simulink model "manning_weir_nonlinear"  (R2022b)
settings: Solver=VariableStepAuto  StartTime=0.0  StopTime=5*N  RelTol=1e-3
libraries: cstblocks x3
settings Model: Creator=chuan  LastModifiedBy=chuan

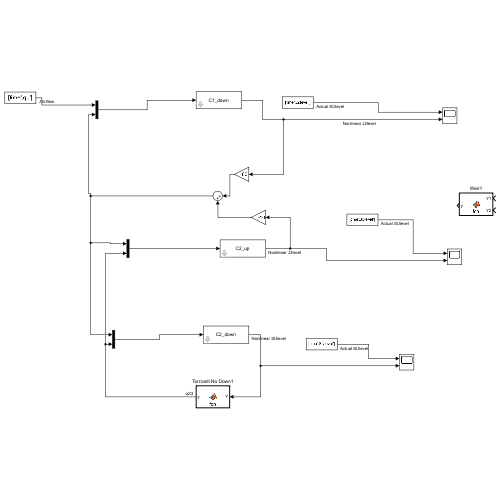
[thumbnail: Simulink's stored preview of the top-level diagram]
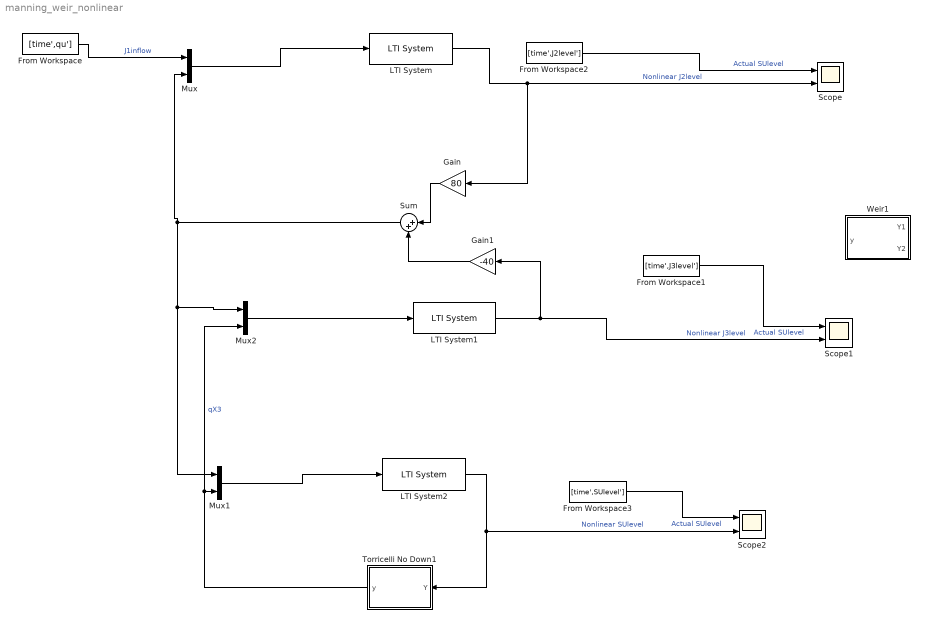
== system manning_weir_nonlinear ==
  From Workspace : FromWorkspace  VariableName=[time',qu']
  From Workspace1 : FromWorkspace  VariableName=[time',J3level']
  From Workspace2 : FromWorkspace  VariableName=[time',J2level']
  From Workspace3 : FromWorkspace  VariableName=[time',SUlevel']
  Gain : Gain  Gain=80
  Gain1 : Gain  Gain=-40
  LTI System : cstblocks/LTI System  sys=C1_down  IC=[]
  LTI System1 : cstblocks/LTI System  sys=C2_up  IC=[]
  LTI System2 : cstblocks/LTI System  sys=C2_down  IC=[]
  Mux : Mux  Inputs=2
  Mux1 : Mux  Inputs=2
  Mux2 : Mux  Inputs=2
  Scope : Scope  NumInputPorts=2
  Scope1 : Scope  NumInputPorts=2
  Scope2 : Scope  NumInputPorts=2
  Sum : Sum  Inputs=|++
  Torricelli No Down1 : MATLAB Function  TreatAsAtomicUnit=on
  Weir1 : MATLAB Function  TreatAsAtomicUnit=on
  wires:
  LTI System/1 -> Gain/1, Scope/2  "Nonlinear J2level"
  Mux/1 -> LTI System/1
  From Workspace/1 -> Mux/1  "J1inflow"
  From Workspace2/1 -> Scope/1  "Actual SUlevel"
  Sum/1 -> Mux/2, Mux2/1, Mux1/1
  Mux1/1 -> LTI System2/1
  LTI System2/1 -> Torricelli No Down1/1(Y), Scope2/2  "Nonlinear SUlevel"
  Torricelli No Down1/1(y) -> Mux2/2, Mux1/2  "qX3"
  Mux2/1 -> LTI System1/1
  LTI System1/1 -> Gain1/1, Scope1/2  "Nonlinear J3level"
  From Workspace1/1 -> Scope1/1  "Actual SUlevel"
  From Workspace3/1 -> Scope2/1  "Actual SUlevel"
  Gain1/1 -> Sum/2
  Gain/1 -> Sum/1

== matlab function manning_weir_nonlinear/Weir1 ==
  data: Y1 input; y output; Y2 input
function y = fcn(Y1,Y2)
Cd = 0.4;
Ws = 10;
Z0 = 1;
g = 9.81;


if Y2 + Z0 >= Ws
    He = Y1-Y2;
    y = Cd*sqrt(2*g)*(He)^(3/2);
else
    He = Y1-Ws;
    He = max(He,0); % if Y1 < Ws, then no flow.
    y = Cd*sqrt(2*g)*(He)^(3/2);
end

== matlab function manning_weir_nonlinear/Torricelli No Down1 ==
  data: Y input; y output
function y = fcn(Y)
Cd = 0.65;
A0 = 100;
g = 9.81;
Z0 = 0;
Yfull = 10;
H_star = Z0 + Yfull;

Y = max(Y,0);
H1 = Y + Z0;

if H1 >= H_star
    He = H1 - (Z0 + Yfull/2);
    y = Cd*A0*sqrt(2*g*He);
else
    CwL = (Cd*A0*sqrt(g))/(Yfull);
    y = CwL*(H1-Z0)^(1.5);
end
